simulink model "NM_Model"  (R2016a)
settings: Solver=ode4  StartTime=0.0  StopTime=TStop  FixedStep=.001  RelTol=1e-3
values from neighbouring files (symbols this model uses):
  Bintrinsic = 5    [Run_NM_Model.m]
  epsi = 1    [Run_NM_Model.m]
  Inertia = 0.005    [Run_NM_Model.m]
  Kintrinsic = 50    [Run_NM_Model.m]
  Kmuscle = 1    [Run_NM_Model.m]
  Kreflex = 50    [Run_NM_Model.m]
  ReflexDelay = .05    (= 0.05)    [Run_NM_Model.m]
  wn = 2*pi    (= 6.28318530718)    [Run_NM_Model.m]
settings Model: Creator=rkearn  LastModifiedBy=rkearn
settings DataIOCC: SaveFormat=Array  SignalLoggingName=sigsOut
settings OptimizationCC: BlockReduction=off  BooleanDataType=off
settings DebuggingCC: SaveWithParameterizedLinksMsg=none  SignalResolutionControl=TryResolveAllWithWarning  MultiTaskDSMMsg=warning  MultiTaskCondExecSysMsg=none  StrictBusMsg=ErrorOnBusTreatedAsVector
settings HardwareCC: ProdBitPerPointer=32  ProdLargestAtomicFloat=None  ProdIntDivRoundTo=Undefined  ProdEndianess=Unspecified  ProdWordSize=32  ProdHWDeviceType=32-bit Generic  TargetBitPerPointer=64  TargetLongLongMode=on  TargetIntDivRoundTo=Zero  TargetEndianess=LittleEndian  TargetWordSize=64  TargetHWDeviceType=MATLAB Host  ProdEqTarget=off
settings ModelReferenceCC: PropagateSignalLabelsOutOfModel=off
settings GRTTargetCC: CombineOutputUpdateFcns=off  GRTInterface=on
settings ConfigComp: CovModelRefEnable=Off

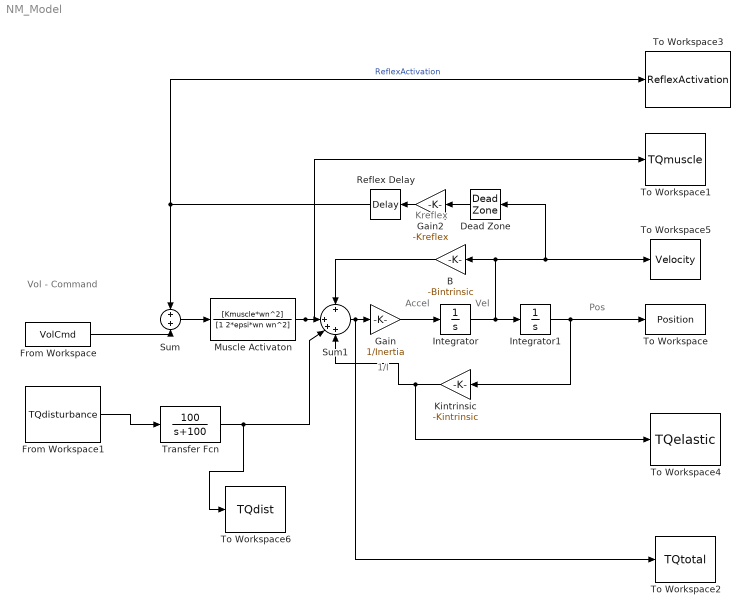
== system NM_Model ==
  note: 1/I
  note: Accel
  note: Vel
  note: Pos
  note: Vol - Command
  note: Kreflex
  B : Gain  Gain=-Bintrinsic  SaturateOnIntegerOverflow=on  OutDataTypeStr=Inherit: Same as input  ParamDataTypeStr=Inherit: Same as input
  Dead Zone : DeadZone  LowerValue=-100  UpperValue=0  SaturateOnIntegerOverflow=on
  From Workspace : FromWorkspace  VariableName=VolCmd  SampleTime=0
  From Workspace1 : FromWorkspace  VariableName=TQdisturbance  SampleTime=0  OutputAfterFinalValue=Setting to zero
  Gain : Gain  Gain=1/Inertia  SaturateOnIntegerOverflow=on  OutDataTypeStr=Inherit: Same as input  ParamDataTypeStr=Inherit: Same as input
  Gain2 : Gain  Gain=-Kreflex  OutDataTypeStr=double  SaturateOnIntegerOverflow=on  ParamDataTypeStr=Inherit: Same as input
  Integrator : Integrator  ContinuousStateAttributes='Velocity'
  Integrator1 : Integrator
  Kintrinsic : Gain  Gain=-Kintrinsic  SaturateOnIntegerOverflow=on  OutDataTypeStr=Inherit: Same as input  ParamDataTypeStr=Inherit: Same as input
  Muscle Activaton : TransferFcn  Numerator=[Kmuscle*wn^2]  Denominator=[1 2*epsi*wn wn^2]
  Reflex Delay : TransportDelay  DelayTime=ReflexDelay  BufferSize=2000
  Sum : Sum  Inputs=2  SaturateOnIntegerOverflow=on  InputSameDT=on  OutDataTypeStr=Inherit: Same as first input
  Sum1 : Sum  Inputs=+|+++  SaturateOnIntegerOverflow=on  InputSameDT=on  OutDataTypeStr=Inherit: Same as first input
  To Workspace : ToWorkspace  VariableName=Position  SaveFormat=Structure With Time  SampleTime=-1
  To Workspace1 : ToWorkspace  VariableName=TQmuscle  SaveFormat=Structure With Time  SampleTime=-1
      settings: Tag=tesat tag
  To Workspace2 : ToWorkspace  VariableName=TQtotal  SaveFormat=Structure With Time  SampleTime=-1
  To Workspace3 : ToWorkspace  VariableName=ReflexActivation  SaveFormat=Structure With Time  SampleTime=-1
  To Workspace4 : ToWorkspace  VariableName=TQelastic  SaveFormat=Structure With Time  SampleTime=-1
  To Workspace5 : ToWorkspace  VariableName=Velocity  SaveFormat=Structure With Time  SampleTime=-1
  To Workspace6 : ToWorkspace  VariableName=TQdist  SaveFormat=Structure With Time  SampleTime=-1
  Transfer Fcn : TransferFcn  Numerator=[100]  Denominator=[1 100]
  wires:
  Integrator/1 -> Dead Zone/1, To Workspace5/1, B/1, Integrator1/1
  Integrator1/1 -> To Workspace/1, Kintrinsic/1
  Gain/1 -> Integrator/1
  Sum/1 -> Muscle Activaton/1
  Gain2/1 -> Reflex Delay/1
  Sum1/1 -> To Workspace2/1, Gain/1
  Reflex Delay/1 -> Sum/1, To Workspace3/1  "ReflexActivation"
  Kintrinsic/1 -> To Workspace4/1, Sum1/4
  B/1 -> Sum1/1
  Muscle Activaton/1 -> Sum1/2, To Workspace1/1
  From Workspace/1 -> Sum/2
  Dead Zone/1 -> Gain2/1
  From Workspace1/1 -> Transfer Fcn/1
  Transfer Fcn/1 -> To Workspace6/1, Sum1/3
